simulink model "SinglePulseModel_n_8"  (R2014a)
settings: Solver=FixedStepDiscrete  StartTime=0.0  StopTime=2000  RelTol=1e-3
InitFcn:
  | initialization;
values from neighbouring files (symbols this model uses):
  delays = tim(T,n,1:n)    [initialization.m]
libraries: BlockLib x26, dspsrcs4 x1
settings Model: Creator=kunalmenda  LastModifiedBy=kunalmenda

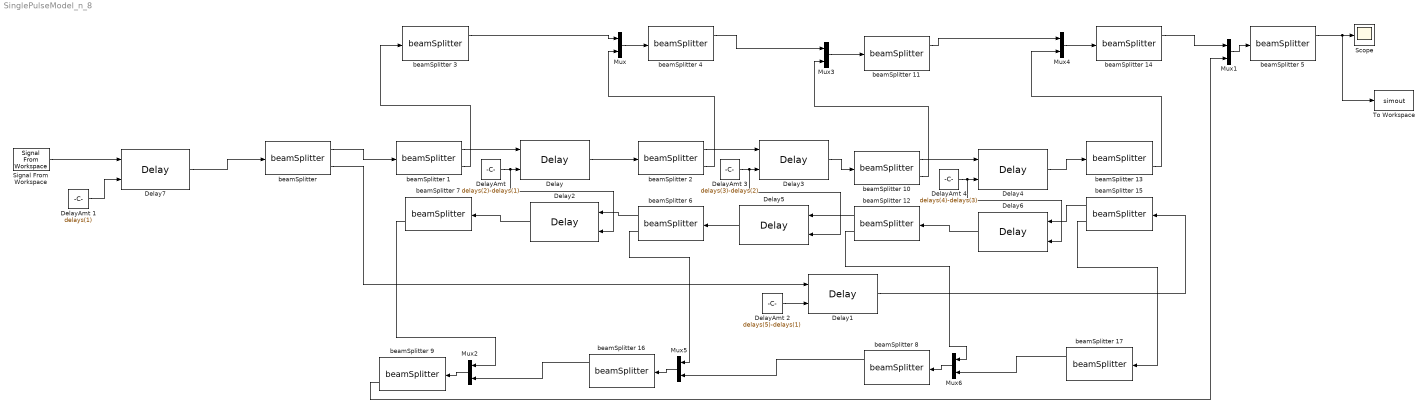
== system SinglePulseModel_n_8 ==
  Delay{,2..7} (7 alike) : BlockLib/Delay
  Delay1 : BlockLib/Delay
      link override Constant: Value=1
  "DelayAmt " : Constant  Value=delays(2)-delays(1)
  DelayAmt 1 : Constant  Value=delays(1)
  DelayAmt 2 : Constant  Value=delays(5)-delays(1)
  DelayAmt 3 : Constant  Value=delays(3)-delays(2)
  DelayAmt 4 : Constant  Value=delays(4)-delays(3)
  Mux{,1..6} (7 alike) : Mux  Inputs=2
  Scope : Scope
  Signal From Workspace : dspsrcs4/Signal From Workspace  X=inputsignal  Ts=1  nsamps=1  OutputAfterFinalValue=Setting to zero  ignoreOrWarnInputAndFrameLengths=off
  To Workspace : ToWorkspace  VariableName=simout  SaveFormat=Timeseries  SampleTime=-1
  beamSplitter {,1..17} (18 alike) : BlockLib/beamSplitter 
  wires:
  "beamSplitter "/1 -> beamSplitter 1/1
  beamSplitter 2/2 -> Mux/2
  beamSplitter 3/1 -> Mux/1
  Mux/1 -> beamSplitter 4/1
  Mux1/1 -> beamSplitter 5/1
  Delay/1 -> beamSplitter 2/1
  beamSplitter 1/2 -> beamSplitter 3/1
  Delay2/1 -> beamSplitter 7/1
  beamSplitter 7/2 -> Mux2/1
  Mux2/1 -> beamSplitter 9/1
  beamSplitter 9/2 -> Mux1/2
  beamSplitter 5/1 -> To Workspace/1, Scope/1
  "beamSplitter "/2 -> Delay1/1
  beamSplitter 1/1 -> Delay/1
  beamSplitter 6/1 -> Delay2/1
  "DelayAmt "/1 -> Delay2/2, Delay/2
  DelayAmt 2/1 -> Delay1/2
  beamSplitter 10/2 -> Mux3/2
  Mux3/1 -> beamSplitter 11/1
  beamSplitter 13/2 -> Mux4/2
  Mux4/1 -> beamSplitter 14/1
  beamSplitter 11/1 -> Mux4/1
  beamSplitter 4/1 -> Mux3/1
  Delay1/1 -> beamSplitter 15/1
  beamSplitter 14/1 -> Mux1/1
  beamSplitter 2/1 -> Delay3/1
  DelayAmt 3/1 -> Delay5/2, Delay3/2
  Delay3/1 -> beamSplitter 10/1
  beamSplitter 10/1 -> Delay4/1
  DelayAmt 4/1 -> Delay6/2, Delay4/2
  Delay4/1 -> beamSplitter 13/1
  beamSplitter 15/1 -> Delay6/1
  Delay6/1 -> beamSplitter 12/1
  beamSplitter 12/1 -> Delay5/1
  Delay5/1 -> beamSplitter 6/1
  Mux5/1 -> beamSplitter 16/1
  beamSplitter 6/2 -> Mux5/1
  Mux6/1 -> beamSplitter 8/1
  beamSplitter 12/2 -> Mux6/1
  beamSplitter 8/1 -> Mux5/2
  beamSplitter 16/1 -> Mux2/2
  beamSplitter 15/2 -> beamSplitter 17/1
  beamSplitter 17/1 -> Mux6/2
  Signal From Workspace/1 -> Delay7/1
  Delay7/1 -> "beamSplitter "/1
  DelayAmt 1/1 -> Delay7/2
